simulink library "driver_model_lib"  (R2022b)
settings: Solver=VariableStepAuto  StartTime=0.0  StopTime=10.0  RelTol=1e-3
settings Model: Creator=dr_pa  LastModifiedBy=dr_pa

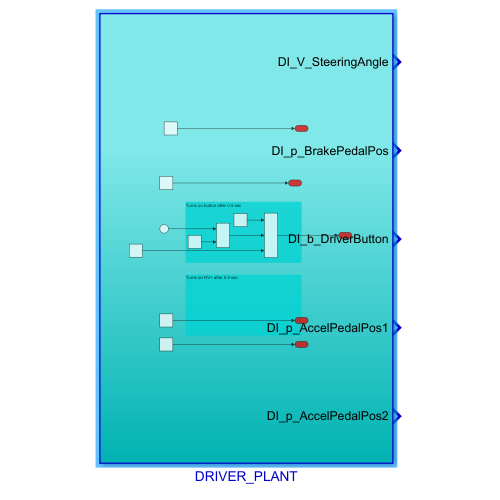
[thumbnail: Simulink's stored preview of the top-level diagram]
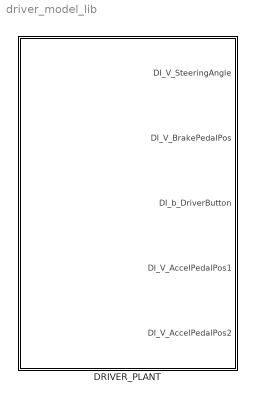
== system driver_model_lib ==
  DRIVER_PLANT : Subsystem

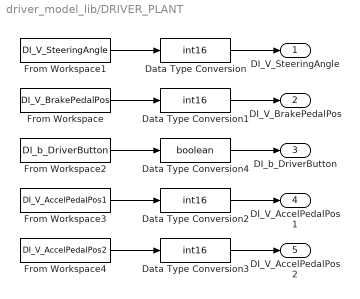
== system driver_model_lib/DRIVER_PLANT ==
  Data Type Conversion{,1..3} (4 alike) : DataTypeConversion  OutDataTypeStr=int16  SaturateOnIntegerOverflow=off  RndMeth=Floor
  Data Type Conversion4 : DataTypeConversion  OutDataTypeStr=boolean  SaturateOnIntegerOverflow=off  RndMeth=Floor
  From Workspace : FromWorkspace  VariableName=DI_V_BrakePedalPos
  From Workspace1 : FromWorkspace  VariableName=DI_V_SteeringAngle
  From Workspace2 : FromWorkspace  VariableName=DI_b_DriverButton
  From Workspace3 : FromWorkspace  VariableName=DI_V_AccelPedalPos1
  From Workspace4 : FromWorkspace  VariableName=DI_V_AccelPedalPos2
  DI_V_SteeringAngle : Outport
  DI_V_BrakePedalPos : Outport  Port=2
  DI_b_DriverButton : Outport  Port=3
  DI_V_AccelPedalPos1 : Outport  Port=4
  DI_V_AccelPedalPos2 : Outport  Port=5
  wires:
  From Workspace/1 -> Data Type Conversion1/1
  From Workspace2/1 -> Data Type Conversion4/1
  From Workspace4/1 -> Data Type Conversion3/1
  From Workspace3/1 -> Data Type Conversion2/1
  From Workspace1/1 -> Data Type Conversion/1
  Data Type Conversion/1 -> DI_V_SteeringAngle/1
  Data Type Conversion4/1 -> DI_b_DriverButton/1
  Data Type Conversion1/1 -> DI_V_BrakePedalPos/1
  Data Type Conversion2/1 -> DI_V_AccelPedalPos1/1
  Data Type Conversion3/1 -> DI_V_AccelPedalPos2/1
